simulink model "Subsystem2"  (R2020b)
settings: Solver=ode15s  StartTime=0.0  StopTime=0.2  RelTol=1e-3
undefined symbols (not defined in the file): b, J, kd, ke, ki, kp, kt, L, R
settings Model: DataDictionary=data_dict.sldd  Creator=Shree  LastModifiedBy=Shree
settings DataIOCC: SaveOutput=off  SaveTime=off

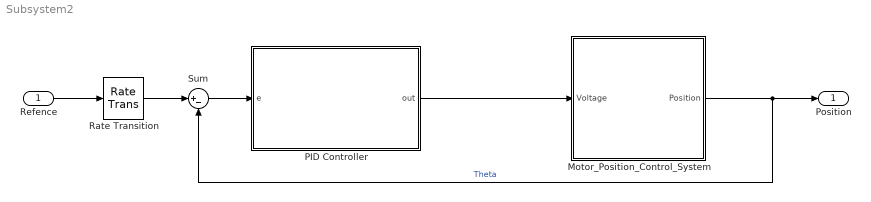
== system Subsystem2 ==
  "Refence " : Inport  OutDataTypeStr=double  PortDimensions=1  SampleTime=[0,1]
  Motor_Position_Control_System : Subsystem
  PID Controller : Subsystem
  Rate Transition : RateTransition
  Sum : Sum  Inputs=|+-
  Position : Outport  OutDataTypeStr=double  PortDimensions=1  SampleTime=0
  wires:
  PID Controller/1(out) -> Motor_Position_Control_System/1(Voltage)
  Motor_Position_Control_System/1(Position) -> Position/1, Sum/2  "Theta"
  Sum/1 -> PID Controller/1(e)
  "Refence "/1 -> Rate Transition/1
  Rate Transition/1 -> Sum/1

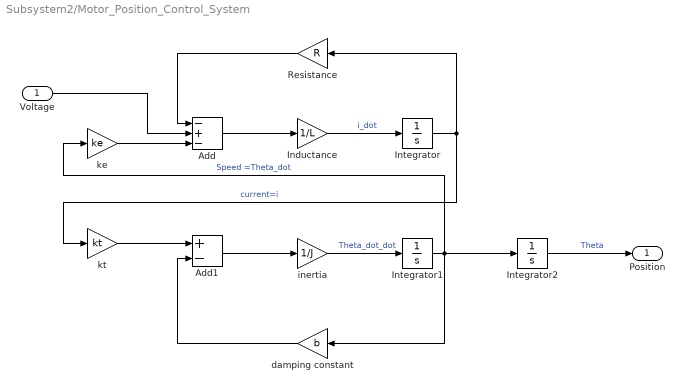
== system Subsystem2/Motor_Position_Control_System ==
  Voltage : Inport
  Add : Sum  Inputs=-+-
  Add1 : Sum  Inputs=+-
  Inductance : Gain  Gain=1/L
  Integrator : Integrator
  Integrator1 : Integrator
  Integrator2 : Integrator
  Resistance : Gain  Gain=R
  damping constant : Gain  Gain=b
  inertia : Gain  Gain=1/J
  ke : Gain  Gain=ke
  kt : Gain  Gain=kt
  Position : Outport
  wires:
  Voltage/1 -> Add/2
  ke/1 -> Add/3
  Integrator2/1 -> Position/1  "Theta"
  Add/1 -> Inductance/1
  damping constant/1 -> Add1/2
  kt/1 -> Add1/1
  Resistance/1 -> Add/1
  Integrator/1 -> kt/1, Resistance/1  "current=i"
  Integrator1/1 -> damping constant/1, ke/1, Integrator2/1  "Speed =Theta_dot"
  Add1/1 -> inertia/1
  inertia/1 -> Integrator1/1  "Theta_dot_dot"
  Inductance/1 -> Integrator/1  "i_dot"

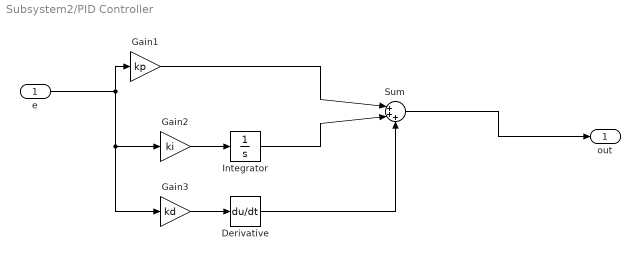
== system Subsystem2/PID Controller ==
  e : Inport
  Derivative : Derivative
  Gain1 : Gain  Gain=kp
  Gain2 : Gain  Gain=ki
  Gain3 : Gain  Gain=kd
  Integrator : Integrator
  Sum : Sum  Inputs=|+++
  out : Outport
  wires:
  Integrator/1 -> Sum/2
  e/1 -> Gain1/1, Gain2/1, Gain3/1
  Sum/1 -> out/1
  Derivative/1 -> Sum/3
  Gain1/1 -> Sum/1
  Gain3/1 -> Derivative/1
  Gain2/1 -> Integrator/1
